simulink model "fullstatefeedback"  (R2023a)
settings: Solver=VariableStepAuto  StartTime=0.0  StopTime=10.0  RelTol=1e-3
values from neighbouring files (symbols this model uses):
  A = [0 0 1 0 0 ... (first row only)    [obsv_ctrb.m]    (also in reduced_order.m = [0 0 1 0)
  B = [0; 0; 0; 0; 1/L_a]    [obsv_ctrb.m]    (also in reduced_order.m = [0; 0; K_m/(J_m * R); 0])
  C = [0 1 0 0 0]    [obsv_ctrb.m]    (also in reduced_order.m = [0 1 0 0]; testobsv.m = [1 0 0 0 0])
  K = place(A, B, p)    [polesplacement.m]
  x1_bar = deg2rad(31.78)    [reduced_order.m]
  x2_bar = deg2rad(30)    [reduced_order.m]
undefined symbols (not defined in the file or in its folder): g, I_noload, init, K_m, l, m, R
settings Model: Creator=yunzh  LastModifiedBy=yunzh

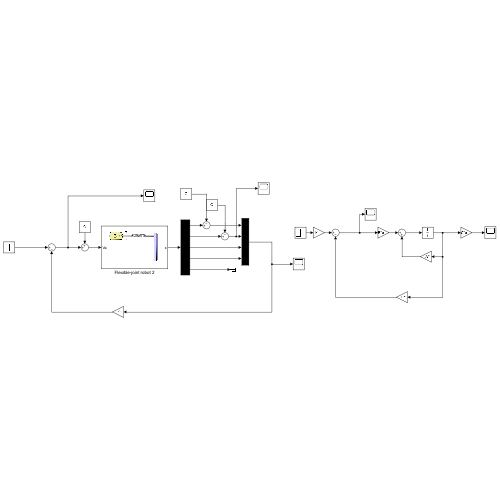
[thumbnail: Simulink's stored preview of the top-level diagram]
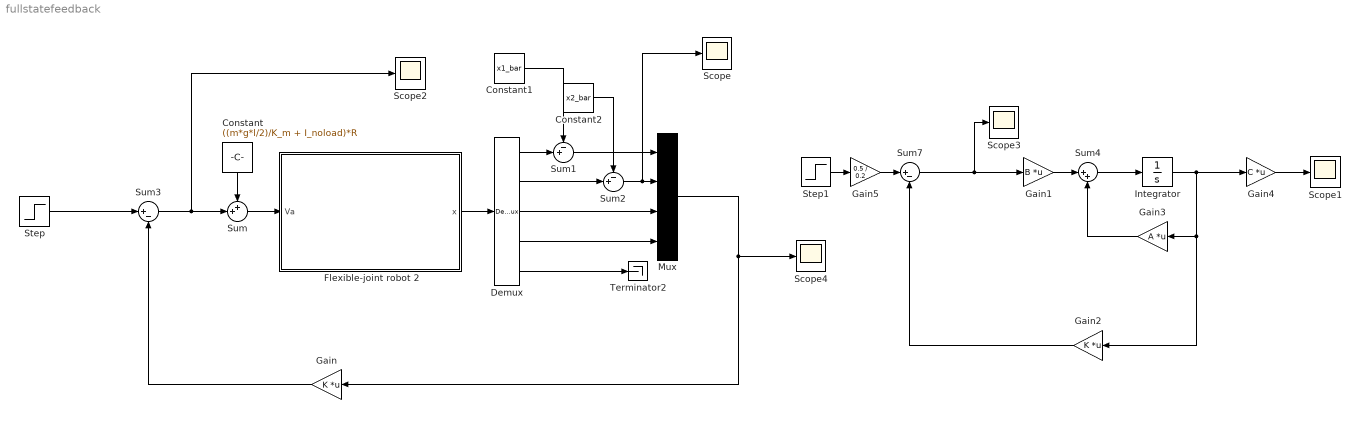
== system fullstatefeedback ==
  Constant : Constant  Value=((m*g*l/2)/K_m + I_noload)*R
  Constant1 : Constant  Value=x1_bar
  Constant2 : Constant  Value=x2_bar
  Demux : Demux  Outputs=5
  Flexible-joint robot 2 : Subsystem
      mask Display: image('$imagefile'); % Use "Edit Image" on toolstrip to change.
  Gain : Gain  Gain=K  Multiplication=Matrix(K*u)
  Gain1 : Gain  Gain=B  Multiplication=Matrix(K*u)
  Gain2 : Gain  Gain=K  Multiplication=Matrix(K*u)
  Gain3 : Gain  Gain=A  Multiplication=Matrix(K*u)
  Gain4 : Gain  Gain=C  Multiplication=Matrix(K*u)
  Gain5 : Gain  Gain=0.5 / 0.2
  Integrator : Integrator
  Mux : Mux
  Scope{,1..4} (5 alike) : Scope
  Step : Step  Time=0  After=0.2  SampleTime=0
  Step1 : Step  Time=0  After=0.5  SampleTime=0
  Sum : Sum  Inputs=++|
  Sum1 : Sum  Inputs=-+|
  Sum2 : Sum  Inputs=-+|
  Sum3 : Sum  Inputs=|+-
  Sum4 : Sum  Inputs=|++
  Sum7 : Sum  Inputs=|+-
  Terminator2 : Terminator
  wires:
  Flexible-joint robot 2/1(x) -> Demux/1
  Sum/1 -> Flexible-joint robot 2/1(Va)
  Demux/4 -> Mux/4
  Demux/3 -> Mux/3
  Mux/1 -> Scope4/1, Gain/1
  Demux/5 -> Terminator2/1
  Demux/1 -> Sum1/2
  Sum1/1 -> Mux/1
  Constant1/1 -> Sum1/1
  Sum2/1 -> Scope/1, Mux/2
  Demux/2 -> Sum2/2
  Constant2/1 -> Sum2/1
  Sum3/1 -> Scope2/1, Sum/2
  Step1/1 -> Gain5/1
  Gain1/1 -> Sum4/1
  Gain3/1 -> Sum4/2
  Sum4/1 -> Integrator/1
  Integrator/1 -> Gain3/1, Gain2/1, Gain4/1
  Gain4/1 -> Scope1/1
  Sum7/1 -> Scope3/1, Gain1/1
  Gain2/1 -> Sum7/2
  Constant/1 -> Sum/1
  Step/1 -> Sum3/1
  Gain5/1 -> Sum7/1
  Gain/1 -> Sum3/2

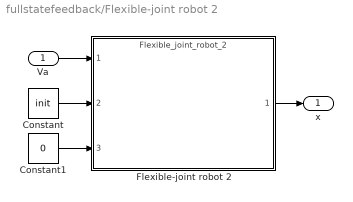
== system fullstatefeedback/Flexible-joint robot 2 ==
  Va : Inport
  Constant : Constant  Value=init
  Constant1 : Constant  Value=0
  Flexible-joint robot 2 : ModelReference  ModelNameDialog=Flexible_joint_robot_2  ModelReferenceVersion=1.65  CopyOfModelProtected=on
  x : Outport
  wires:
  Va/1 -> Flexible-joint robot 2/1
  Constant1/1 -> Flexible-joint robot 2/3
  Constant/1 -> Flexible-joint robot 2/2
  Flexible-joint robot 2/1 -> x/1
